simulink model "Visualization_2DPointMass"  (R2018b)
settings: Solver=FixedStepAuto  StartTime=0.0  StopTime=EndTime  FixedStep=h  MaxStep=0.001  RelTol=1e-6  EnableMultiTasking=on
values from neighbouring files (symbols this model uses):
  FFx_result = result.x(find(names == 'FFx0'):find(names == FFx_label(end)))    [MAIN.m]    (also in good_result_show_angular_momentum_knitro.mat = [219.331381652 0 14.0569251132 -55.7169525245 0 0 -79.059425; samll_example_success_Knitro.mat = [299.999991306 0 0 0 0 0 0 0 0 -299.999868357 3.08050382687e; very beautiful result non-sparse Q.mat = [173.076866714 154.411687669 0 0 0 0 0 0 0 0 0 -32.239846101; very beautiful result sparse Q.mat = [144.164781547 128.718575206 0 0 0 0 0 0 20.5946289574 0 0 0)
  FFy_result = result.x(find(names == 'FFy0'):find(names == FFy_label(end)))    [MAIN.m]    (also in good_result_show_angular_momentum_knitro.mat = [258.165846204 0 293.511156735 348.245408 0 0 438.434174007 ; samll_example_success_Knitro.mat = [702.906217002 0 0 0 0 0 0 0 0 1596.49513821 0.0060476997901; very beautiful result non-sparse Q.mat = [763.787177034 767.947229012 0 0 0 0 0 0 0 0 0 809.547825632; very beautiful result sparse Q.mat = [711.935819151 714.460408289 0 0 0 0 0 0 732.132759792 0 0 0)
  FHx_result = result.x(find(names == 'FHx0'):find(names == FHx_label(end)))    [MAIN.m]    (also in good_result_show_angular_momentum_knitro.mat = [219.331741842 89.1008749223 0 0 0 0 -79.0596647203 0 41.812; samll_example_success_Knitro.mat = [300.000008694 0 0 0 0 0 0 0 0 -300.000131643 3.07593421777e; very beautiful result non-sparse Q.mat = [173.076921264 0 0 0 0 79.7510700195 0 0 0 5.090981472 0 -32; very beautiful result sparse Q.mat = [144.164862247 0 113.272369877 0 0 0 0 0 20.5949514338 0 0 -)
  FHy_result = result.x(find(names == 'FHy0'):find(names == FHy_label(end)))    [MAIN.m]    (also in good_result_show_angular_momentum_knitro.mat = [971.03554966 926.236054705 0 0 0 0 703.173687604 0 608.0526; samll_example_success_Knitro.mat = [1503.590033 0 0 0 0 0 0 0 0 610.001111786 0.00779775057198]; very beautiful result non-sparse Q.mat = [763.787140899 0 0 0 0 784.587479326 0 0 0 801.227716233 0 8; very beautiful result sparse Q.mat = [711.935879282 0 716.98503127 0 0 0 0 0 732.132636773 0 0 73)
  I = 2.1    [MAIN.m]    (also in good_result_show_angular_momentum_knitro.mat; samll_example_success_Knitro.mat; very beautiful result non-sparse Q.mat; very beautiful result sparse Q.mat)
  m = 45    [MAIN.m]    (also in good_result_show_angular_momentum_knitro.mat; samll_example_success_Knitro.mat; very beautiful result non-sparse Q.mat; very beautiful result sparse Q.mat)
  PFx_result = result.x(find(names == 'PFx0'):find(names == PFx_label(end)))    [MAIN.m]    (also in very beautiful result non-sparse Q.mat = [0.171137629229 0.171137629229 0.171137629229 0.233713576151; very beautiful result sparse Q.mat = [0.183977613483 0.183977613483 0.183977613483 0.247848791945; very beautiful sparse solution.mat = [0.189943267114 0.189943267114 0.189943267114 0.189943267114)
  PFy_result = result.x(find(names == 'PFy0'):find(names == PFy_label(end)))    [MAIN.m]    (also in very beautiful result non-sparse Q.mat = [0 0 0 0.0705134606984 0.130151077634 0.177427787359 0.20981; very beautiful result sparse Q.mat = [0 0 0 0.0585810398512 0.0911836476563 0.105739546433 0.1060; very beautiful sparse solution.mat = [0 0 0 0 0.0504729097199 0.0708917537602 0 0 0 0 0.136609496)
  PHx_result = result.x(find(names == 'PHx0'):find(names == PHx_label(end)))    [MAIN.m]    (also in very beautiful result non-sparse Q.mat = [-0.333853990809 -0.333853990809 -0.267581905843 -0.22180938; very beautiful result sparse Q.mat = [-0.315273330446 -0.315273330446 -0.253339698875 -0.25333969; very beautiful sparse solution.mat = [-0.272858093752 -0.272858093752 -0.272858093752 -0.27285809)
  PHy_result = result.x(find(names == 'PHy0'):find(names == PHy_label(end)))    [MAIN.m]    (also in very beautiful result non-sparse Q.mat = [0 0 0.0360195691746 0.0510079153443 0.0486299033838 0 0 0.0; very beautiful result sparse Q.mat = [0 0 0 0 0.0578623291222 0.0887165243176 0.0924186256593 0.0; very beautiful sparse solution.mat = [0 0 0 0 0 0 0 0 0 0 0 0 ... (21 elements, 21x1)])
  TimeSeries = 0:h:EndTime    [MAIN.m]    (also in good_result_show_angular_momentum_knitro.mat = [0 0.05 0.1 0.15 0.2 0.25 0.3 0.35 0.4 0.45 0.5 0.55 ... (21; samll_example_success_Knitro.mat = [0 0.05 0.1 0.15 0.2 0.25 0.3 0.35 0.4 0.45 0.5]; very beautiful result non-sparse Q.mat = [0 0.05 0.1 0.15 0.2 0.25 0.3 0.35 0.4 0.45 0.5 0.55 ... (21; very beautiful result sparse Q.mat = [0 0.05 0.1 0.15 0.2 0.25 0.3 0.35 0.4 0.45 0.5 0.55 ... (21)
  x_result = result.x(find(names == 'x0'):find(names == x_label(end)))    [MAIN.m]    (also in very beautiful result non-sparse Q.mat = [0 3.68944102897e-21 0.0192307659988 0.0470399590902 0.07484; very beautiful result sparse Q.mat = [0 0 0.0160183135441 0.039187659044 0.0686499139816 0.098112; very beautiful sparse solution.mat = [0 1.6731499127e-14 0.0101928934712 0.0293730757838 0.056334)
  y_result = result.x(find(names == 'y0'):find(names == y_label(end)))    [MAIN.m]    (also in very beautiful result non-sparse Q.mat = [0.3 0.3 0.360348614885 0.438844339715 0.492823439546 0.5222; very beautiful result sparse Q.mat = [0.3 0.3 0.354587358246 0.424350336397 0.509429191286 0.5699; very beautiful sparse solution.mat = [0.3 0.3 0.30960888592 0.330062696666 0.362597473019 0.37061)
libraries: nesl_utility x12, sm_lib x4
settings Model: Creator=jiayu  LastModifiedBy=jiayu
settings DataIOCC: LimitDataPoints=on
settings OptimizationCC: LifeSpan=inf
settings DebuggingCC: AllowSymbolicDim=off  SFUnexpectedBacktrackingDiag=warning  SFNoUnconditionalDefaultTransitionDiag=warning  SFExecutionAtInitializationDiag=none
settings SFSimCC: SimUseLocalCustomCode=off
settings RTWCC: RTWUseLocalCustomCode=off
settings CodeAppCC: StateflowObjectComments=on
settings GRTTargetCC: TargetLangStandard=C89/C90 (ANSI)  GeneratePreprocessorConditionals=Disable all
settings ConfigComp: CovMetricSettings=dw  CovHtmlReporting=on  CovSaveCumulativeToWorkspaceVar=on  CovSaveSingleToWorkspaceVar=on  CovExternalEMLEnable=off  CovSFcnEnable=off
settings SimscapeCC: SimscapeNominalValues="[{\"value\":\"10\",\"unit\":\"V\"},{\"value\":\"1\",\"unit\":\"A\"},{\"value\":\"10\",\"unit\":\"N*m\"},{\"value\":\"10\",\"unit\":\"bar\"},{\"value\":\"100\",\"unit\":\"kJ/kg\"},{\"value\":\"1\",\"unit\":\"kW\"},{\"value\":\"300\",\"unit\":\"K\"},{\"value\":\"100\",\"unit\":\"cm^3/s\"},{\"value\":\"1\",\"unit\":\"kN\"},{\"value\":\"1\",\"unit\":\"g/cm^3\"},{\"value\":\"1\",\"unit\":\"l\"},{\"value\":\"1\",\"unit\":\"cm^2\"},{\"value\":\"60\",\"unit\":\"Hz\"}]"  SimscapeLogType=all  SimscapeLogDataHistory=10000
settings ConfigurationSet: Description=SimMechanics 2G

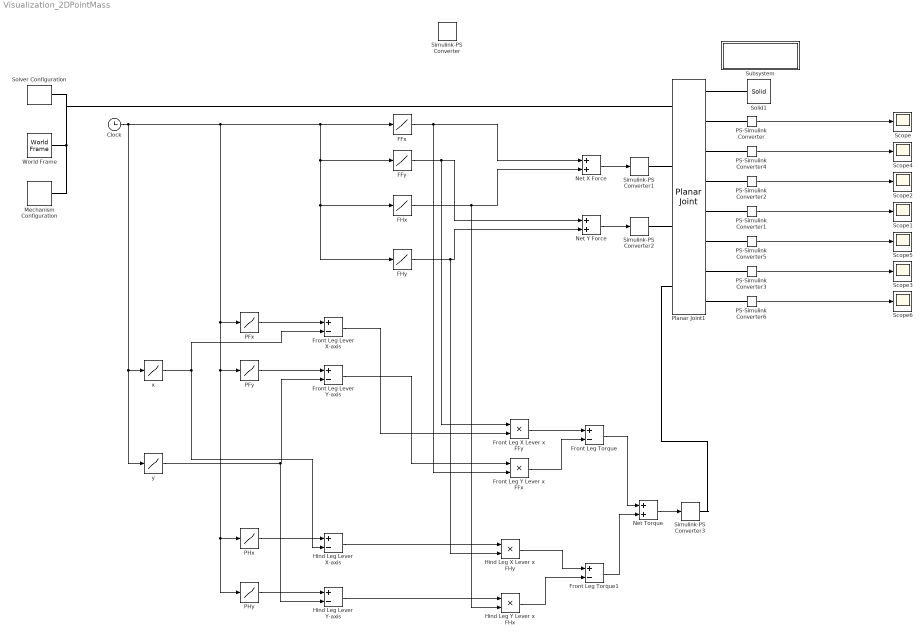
== system Visualization_2DPointMass ==
  Clock : Clock
  FFx : Lookup_n-D  NumberOfTableDimensions=1  BreakpointsForDimension1=TimeSeries  Table=FFx_result  InterpMethod=Flat  InternalRulePriority=Speed  RndMeth=Simplest  InputSameDT=on
  FFy : Lookup_n-D  NumberOfTableDimensions=1  BreakpointsForDimension1=TimeSeries  Table=FFy_result  InterpMethod=Flat  InternalRulePriority=Speed  RndMeth=Simplest  InputSameDT=on
  FHx : Lookup_n-D  NumberOfTableDimensions=1  BreakpointsForDimension1=TimeSeries  Table=FHx_result  InterpMethod=Flat  InternalRulePriority=Speed  RndMeth=Simplest  InputSameDT=on
  FHy : Lookup_n-D  NumberOfTableDimensions=1  BreakpointsForDimension1=TimeSeries  Table=FHy_result  InterpMethod=Flat  InternalRulePriority=Speed  RndMeth=Simplest  InputSameDT=on
  Front Leg Lever X-axis : Sum  Inputs=+-
  Front Leg Lever Y-axis : Sum  Inputs=+-
  Front Leg Torque : Sum  Inputs=+-
  Front Leg Torque1 : Sum  Inputs=+-
  Front Leg X Lever x FFy : Product
  Front Leg Y Lever x FFx : Product
  Hind Leg Lever X-axis : Sum  Inputs=+-
  Hind Leg Lever Y-axis : Sum  Inputs=+-
  Hind Leg X Lever x FHy : Product
  Hind Leg Y Lever x FHx : Product
  Mechanism Configuration : sm_lib/Utilities/Mechanism Configuration  UniformGravity=Constant  GravityVector=[0 -9.80665 0]  GravityUnits=m/s^2  LinearizationDelta=0.001
  Net Torque : Sum
  Net X Force : Sum
  Net Y Force : Sum
  PFx : Lookup_n-D  NumberOfTableDimensions=1  BreakpointsForDimension1=TimeSeries  Table=PFx_result  InterpMethod=Flat  InternalRulePriority=Speed  RndMeth=Simplest  InputSameDT=on
  PFy : Lookup_n-D  NumberOfTableDimensions=1  BreakpointsForDimension1=TimeSeries  Table=PFy_result  InterpMethod=Flat  InternalRulePriority=Speed  RndMeth=Simplest  InputSameDT=on
  PHx : Lookup_n-D  NumberOfTableDimensions=1  BreakpointsForDimension1=TimeSeries  Table=PHx_result  InterpMethod=Flat  InternalRulePriority=Speed  RndMeth=Simplest  InputSameDT=on
  PHy : Lookup_n-D  NumberOfTableDimensions=1  BreakpointsForDimension1=TimeSeries  Table=PHy_result  InterpMethod=Flat  InternalRulePriority=Speed  RndMeth=Simplest  InputSameDT=on
  PS-Simulink Converter : nesl_utility/PS-Simulink Converter  PhysicalDomain=network_engine_domain  SubClassName=ps_output  LeftPortType=input  RightPortType=output  PseudoPeriodic=off  Frequencies=[]  Unit=m  AffineConversion=off
  PS-Simulink Converter1 : nesl_utility/PS-Simulink Converter  PhysicalDomain=network_engine_domain  SubClassName=ps_output  LeftPortType=input  RightPortType=output  PseudoPeriodic=off  Frequencies=[]  Unit=m  AffineConversion=off
  PS-Simulink Converter2 : nesl_utility/PS-Simulink Converter  PhysicalDomain=network_engine_domain  SubClassName=ps_output  LeftPortType=input  RightPortType=output  PseudoPeriodic=off  Frequencies=[]  Unit=N  AffineConversion=off
  PS-Simulink Converter3 : nesl_utility/PS-Simulink Converter  PhysicalDomain=network_engine_domain  SubClassName=ps_output  LeftPortType=input  RightPortType=output  PseudoPeriodic=off  Frequencies=[]  Unit=N  AffineConversion=off
  PS-Simulink Converter4 : nesl_utility/PS-Simulink Converter  PhysicalDomain=network_engine_domain  SubClassName=ps_output  LeftPortType=input  RightPortType=output  PseudoPeriodic=off  Frequencies=[]  Unit=m/s  AffineConversion=off
  PS-Simulink Converter5 : nesl_utility/PS-Simulink Converter  PhysicalDomain=network_engine_domain  SubClassName=ps_output  LeftPortType=input  RightPortType=output  PseudoPeriodic=off  Frequencies=[]  Unit=m/s  AffineConversion=off
  PS-Simulink Converter6 : nesl_utility/PS-Simulink Converter  PhysicalDomain=network_engine_domain  SubClassName=ps_output  LeftPortType=input  RightPortType=output  PseudoPeriodic=off  Frequencies=[]  Unit=rad  AffineConversion=off
  Planar Joint1 : sm_lib/Joints/Planar Joint  SenseConstraintForce=off  SenseConstraintForceX=off  SenseConstraintForceY=off  SenseConstraintForceZ=off  SenseConstraintTorque=off  SenseConstraintTorqueX=off  SenseConstraintTorqueY=off  SenseConstraintTorqueZ=off  SenseTotalForce=off  SenseTotalForceX=off  SenseTotalForceY=off  SenseTotalForceZ=off  SenseTotalTorque=off  SenseTotalTorqueX=off  SenseTotalTorqueY=off  SenseTotalTorqueZ=off  CompositeWrenchDir=FollowerOnBase  CompositeWrenchFrame=BaseFrame  PxEquilibriumPosition=0  PxEquilibriumPositionUnits=m  PxSpringStiffness=0  PxSpringStiffnessUnits=N/m  PxDampingCoefficient=0  PxDampingCoefficientUnits=N/(m/s)  PxTorqueActuationMode=InputTorque  PxMotionActuationMode=ComputedMotion  PxSensePosition=on  PxSenseVelocity=on  PxSenseAcceleration=off  PxSenseTorqueForce=on  PxPositionTargetSpecify=on  PxPositionTargetPriority=High  PxPositionTargetValue=x_init  PxPositionTargetValueUnits=m  PxVelocityTargetSpecify=on  PxVelocityTargetPriority=High  PxVelocityTargetValue=0  PxVelocityTargetValueUnits=m/s  PyEquilibriumPosition=0  PyEquilibriumPositionUnits=m  PySpringStiffness=0  PySpringStiffnessUnits=N/m  PyDampingCoefficient=0  PyDampingCoefficientUnits=N/(m/s)  PyTorqueActuationMode=InputTorque  PyMotionActuationMode=ComputedMotion  PySensePosition=on  PySenseVelocity=on  PySenseAcceleration=off  PySenseTorqueForce=on  PyPositionTargetSpecify=on  PyPositionTargetPriority=High  PyPositionTargetValue=y_init  PyPositionTargetValueUnits=m  PyVelocityTargetSpecify=off  PyVelocityTargetPriority=High  PyVelocityTargetValue=0  PyVelocityTargetValueUnits=m/s  RzEquilibriumPosition=0  RzEquilibriumPositionUnits=deg  RzSpringStiffness=0  RzSpringStiffnessUnits=N*m/deg  RzDampingCoefficient=0  RzDampingCoefficientUnits=N*m/(deg/s)  RzTorqueActuationMode=InputTorque  RzMotionActuationMode=ComputedMotion  RzSensePosition=on  RzSenseVelocity=off  RzSenseAcceleration=off  RzSenseTorqueForce=off  RzPositionTargetSpecify=on  RzPositionTargetPriority=High  RzPositionTargetValue=0  RzPositionTargetValueUnits=deg  RzVelocityTargetSpecify=on  RzVelocityTargetPriority=High  RzVelocityTargetValue=0  RzVelocityTargetValueUnits=deg/s
  Scope{,1..6} (7 alike) : Scope
  Simulink-PS Converter : nesl_utility/Simulink-PS Converter  PhysicalDomain=network_engine_domain  SubClassName=ps_input  LeftPortType=input  RightPortType=output  PseudoPeriodic=off  Frequencies=[]  NoiseDistribution=none  NoiseParameters=[]  Unit=1  AffineConversion=off  FilteringAndDerivatives=zero  SimscapeFilterOrder=1  InputFilterTimeConstant=0.001  UdotUserProvided=1
  Simulink-PS Converter1 : nesl_utility/Simulink-PS Converter  PhysicalDomain=network_engine_domain  SubClassName=ps_input  LeftPortType=input  RightPortType=output  PseudoPeriodic=off  Frequencies=[]  NoiseDistribution=none  NoiseParameters=[]  Unit=N  AffineConversion=off  FilteringAndDerivatives=zero  SimscapeFilterOrder=1  InputFilterTimeConstant=0.001  UdotUserProvided=1
  Simulink-PS Converter2 : nesl_utility/Simulink-PS Converter  PhysicalDomain=network_engine_domain  SubClassName=ps_input  LeftPortType=input  RightPortType=output  PseudoPeriodic=off  Frequencies=[]  NoiseDistribution=none  NoiseParameters=[]  Unit=N  AffineConversion=off  FilteringAndDerivatives=zero  SimscapeFilterOrder=1  InputFilterTimeConstant=0.001  UdotUserProvided=1
  Simulink-PS Converter3 : nesl_utility/Simulink-PS Converter  PhysicalDomain=network_engine_domain  SubClassName=ps_input  LeftPortType=input  RightPortType=output  PseudoPeriodic=off  Frequencies=[]  NoiseDistribution=none  NoiseParameters=[]  Unit=N*m  AffineConversion=off  FilteringAndDerivatives=zero  SimscapeFilterOrder=1  InputFilterTimeConstant=0.001  UdotUserProvided=1
  Solid1 : sm_lib/Body Elements/Solid  InertiaType=Custom  Mass=m  MassUnits=kg  CenterOfMass=[0 0 0]  CenterOfMassUnits=m  MomentsOfInertia=[0.35 I I]  MomentsOfInertiaUnits=kg*m^2  ProductsOfInertia=[0 0 0]  ProductsOfInertiaUnits=kg*m^2  BasedOnType=Mass  Density=1000  DensityUnits=kg/m^3  DoExposeReferenceFrame=on  SerializedFrames=<Frames/>  GraphicType=FromGeometry  MarkerShape=Sphere  MarkerSize=10  GraphicVisPropType=SimpleVisualProperties  GraphicDiffuseColor=[1.0 0.2 0.2]  GraphicSpecularColor=[0.5 0.5 0.5 1.0]  GraphicAmbientColor=[0.15 0.15 0.15 1.0]  GraphicEmissiveColor=[0.0 0.0 0.0 1.0]  GraphicShininess=75  GraphicOpacity=1.0  GeometryShape=Brick  RectangleSize=[1 1]  RectangleSizeUnits=m  BrickDimensions=[0.6 0.256 0.2]  BrickDimensionUnits=m  CylinderRadius=1  CylinderRadiusUnits=m  CylinderLength=1  CylinderLengthUnits=m  SphereRadius=1  SphereRadiusUnits=m  EllipsoidRadii=[1 1 1]  EllipsoidRadiiUnits=m  ExtrusionCrossSection=[1 1; -1 1; -1 -1; 1 -1]  ExtrusionCrossSectionUnits=m  ExtrusionLength=1  ExtrusionLengthUnits=m  PolygonNumSides=3  PolygonOuterRadius=1  PolygonOuterRadiusUnits=m  ExtGeomFileType=STEP  ExtGeomFileUnits=m  RevolutionCrossSection=[1 1; 1 -1; 2 -1; 2 1]  RevolutionCrossSectionUnits=m  RevolutionExtent=Full  RevolutionAngle=180  RevolutionAngleUnits=deg
  Solver Configuration : nesl_utility/Solver Configuration  PhysicalDomain=network_engine_domain  SubClassName=solver  LeftPortType=input  RightPortType=generic  Tones=[]  Harmonics=[]  SimulateNoise=off  Profile=off  UseLocalSampling=off  EnableSwitchedLinearOptims=on  FrequencyDomain=off  UseCCode=off  RelTol=0.001  AbsTol=1e-06  MinStep=1e-09  ToWorkspace=off  RevertToSquareIcSolve=off  NumHomotopyIterations=100  PhasorMode=off  PhasorModeNumHarmonics=1  DoDC=off  ResidualTolerance=1e-09  UseLocalSolver=off  LocalSolverChoice=NE_BACKWARD_EULER_ADVANCER  LocalSolverSampleTime=0.001  DoFixedCost=off  MaxNonlinIter=3  MaxModeIter=2  LinearAlgebra=Sparse  EquationFormulation=NE_TIME_EF  DelaysMemoryBudget=1024  AutomaticFiltering=on  FilteringTimeConstant=0.001  PartitionStorageMethod=AS_NEEDED  PartitionMemoryBudget=1024
  Subsystem : Subsystem
      settings: OpenFcn=open_system('sm_lib')
      mask Display: disp(sprintf('Open Simscape Multibody\nLibrary'));
  World Frame : sm_lib/Frames and Transforms/World Frame
  x : Lookup_n-D  NumberOfTableDimensions=1  BreakpointsForDimension1=TimeSeries  Table=x_result  InterpMethod=Flat  InternalRulePriority=Speed  RndMeth=Simplest  InputSameDT=on
  y : Lookup_n-D  NumberOfTableDimensions=1  BreakpointsForDimension1=TimeSeries  Table=y_result  InterpMethod=Flat  InternalRulePriority=Speed  RndMeth=Simplest  InputSameDT=on
  wires:
  Net X Force/1 -> Simulink-PS Converter1/1
  Net Y Force/1 -> Simulink-PS Converter2/1
  FFx/1 -> Front Leg Y Lever x FFx/2, Net X Force/1
  FHx/1 -> Hind Leg Y Lever x FHx/2, Net X Force/2
  FFy/1 -> Front Leg X Lever x FFy/1, Net Y Force/1
  FHy/1 -> Hind Leg X Lever x FHy/2, Net Y Force/2
  Clock/1 -> y/1, x/1, PHy/1, PHx/1, PFy/1, PFx/1, FHy/1, FHx/1, FFy/1, FFx/1
  PFx/1 -> Front Leg Lever X-axis/1
  PS-Simulink Converter/1 -> Scope/1
  PFy/1 -> Front Leg Lever Y-axis/1
  PS-Simulink Converter1/1 -> Scope1/1
  PHx/1 -> Hind Leg Lever X-axis/1
  PHy/1 -> Hind Leg Lever Y-axis/1
  Front Leg Lever X-axis/1 -> Front Leg X Lever x FFy/2
  Front Leg Lever Y-axis/1 -> Front Leg Y Lever x FFx/1
  Front Leg X Lever x FFy/1 -> Front Leg Torque/1
  Front Leg Y Lever x FFx/1 -> Front Leg Torque/2
  Front Leg Torque/1 -> Net Torque/1
  Hind Leg Lever X-axis/1 -> Hind Leg X Lever x FHy/1
  Hind Leg Lever Y-axis/1 -> Hind Leg Y Lever x FHx/1
  Hind Leg X Lever x FHy/1 -> Front Leg Torque1/1
  Hind Leg Y Lever x FHx/1 -> Front Leg Torque1/2
  Front Leg Torque1/1 -> Net Torque/2
  Net Torque/1 -> Simulink-PS Converter3/1
  PS-Simulink Converter4/1 -> Scope4/1
  PS-Simulink Converter2/1 -> Scope2/1
  PS-Simulink Converter5/1 -> Scope5/1
  PS-Simulink Converter3/1 -> Scope3/1
  PS-Simulink Converter6/1 -> Scope6/1
  x/1 -> Hind Leg Lever X-axis/2, Front Leg Lever X-axis/2
  y/1 -> Hind Leg Lever Y-axis/2, Front Leg Lever Y-axis/2
  connections:
  Mechanism Configuration/RConn1 -- Solver Configuration/RConn1 -- Planar Joint1/LConn1 -- World Frame/RConn1
  Solid1/RConn1 -- Planar Joint1/RConn1
  Simulink-PS Converter1/RConn1 -- Planar Joint1/LConn2
  Simulink-PS Converter2/RConn1 -- Planar Joint1/LConn3
  Planar Joint1/RConn3 -- PS-Simulink Converter4/LConn1
  PS-Simulink Converter5/LConn1 -- Planar Joint1/RConn6
  PS-Simulink Converter/LConn1 -- Planar Joint1/RConn2
  PS-Simulink Converter2/LConn1 -- Planar Joint1/RConn4
  Planar Joint1/RConn5 -- PS-Simulink Converter1/LConn1
  PS-Simulink Converter3/LConn1 -- Planar Joint1/RConn7
  PS-Simulink Converter6/LConn1 -- Planar Joint1/RConn8
  Simulink-PS Converter3/RConn1 -- Planar Joint1/LConn4

== system Visualization_2DPointMass/Subsystem ==
